simulink model "final"  (R2017b)
settings: Solver=VariableStepAuto  StartTime=0.0  StopTime=10.0  RelTol=1e-3
settings Model: Creator=Sofia  LastModifiedBy=Sofia

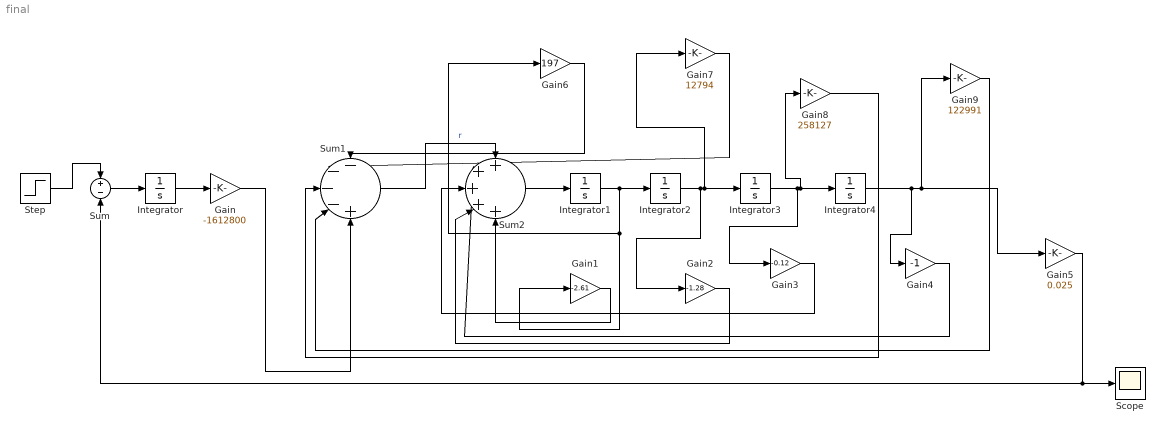
== system final ==
  Gain : Gain  Gain=-1612800
  Gain1 : Gain  Gain=-2.61
  Gain2 : Gain  Gain=-1.28
  Gain3 : Gain  Gain=-0.12
  Gain4 : Gain  Gain=-1
  Gain5 : Gain  Gain=0.025
  Gain6 : Gain  Gain=197
  Gain7 : Gain  Gain=12794
  Gain8 : Gain  Gain=258127
  Gain9 : Gain  Gain=122991
  Integrator{,1..4} (5 alike) : Integrator
  Scope : Scope
  Step : Step  SampleTime=0
  Sum : Sum  Inputs=+-
  Sum1 : Sum  Inputs=----+
  Sum2 : Sum  Inputs=+++++
  wires:
  Step/1 -> Sum/1
  Sum/1 -> Integrator/1
  Gain5/1 -> Scope/1, Sum/2
  Integrator/1 -> Gain/1
  Gain/1 -> Sum1/5
  Sum2/1 -> Integrator1/1
  Integrator1/1 -> Gain6/1, Gain1/1, Integrator2/1
  Integrator2/1 -> Gain2/1, Gain7/1, Integrator3/1
  Integrator3/1 -> Gain3/1, Gain8/1, Integrator4/1
  Sum1/1 -> Sum2/1  "r"
  Gain1/1 -> Sum2/5
  Gain2/1 -> Sum2/4
  Gain3/1 -> Sum2/3
  Integrator4/1 -> Gain9/1, Gain5/1, Gain4/1
  Gain4/1 -> Sum2/2
  Gain6/1 -> Sum1/1
  Gain7/1 -> Sum1/2
  Gain8/1 -> Sum1/3
  Gain9/1 -> Sum1/4
